simulink model "FSM"  (R2024b)
settings: Solver=VariableStepAuto  StartTime=0.0  StopTime=10.0  RelTol=1e-3
settings Model: Creator=leon-  LastModifiedBy=leon-

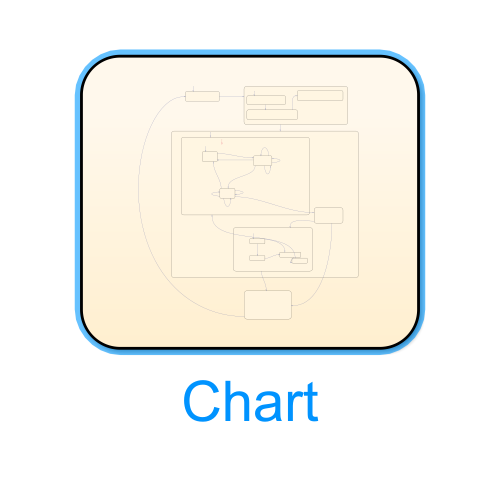
[thumbnail: Simulink's stored preview of the top-level diagram]
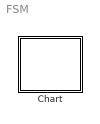
== system FSM ==
  Chart : Stateflow chart  TreatAsAtomicUnit=on

== stateflow chart FSM/Chart ==
  state Difficulty_Selection
    state Selected_Difficulty
      display_line1 = 'Selected Diff:';
      display_line2 = ['Level: ' num2str(difficulty_value)];
    state Inital_Difficulty
      display_line1 = "Difficuly";
      display_line2 = "Selection";
    state Change_Difficulty
      display_line1 = "Press Red: Change";
      display_line2 = "Press Blue: Start";
    (default) -> Inital_Difficulty : {timer = 0}
    Change_Difficulty -> Selected_Difficulty : [red_button]{changeLevel()}
    Inital_Difficulty -> Change_Difficulty : [timer > 3]
  state Idle
    display_line1="Reload and Press";
    display_line2="Button to Start";
  state In_Game
    state Human_Turn
      display_line1 = "Waiting for";
      display_line2 = "your Move";
      state Initial_IR
      state Triggered_IR
        triggered_IR = IR;
      state Wait_IR
      (default) -> Initial_IR
      Triggered_IR -> Triggered_IR [order 2] : [IR~=triggered_IR && ~timer_2]{timer_2 = 0}
      Initial_IR -> Triggered_IR : [IR]{timer_1 = 0}
      Triggered_IR -> Triggered_IR [order 4] : [IR~=triggered_IR && timer_2<0.01]
      Triggered_IR -> Initial_IR [order 1] : [IR~=triggered_IR] && timer_2=>0.01
      Wait_IR -> Initial_IR [order 3] : [IR~=triggered_IR] && timer_2=>0.01
      Triggered_IR -> Wait_IR [order 3] : [timer_1 > 0.02]{timer_1 = 0}
      Triggered_IR -> Triggered_IR [order 5] : [IR == triggered_IR]{~timer_2}
      Wait_IR -> Wait_IR [order 1] : [IR~=triggered_IR && ~timer_2]{timer_2 = 0}
      Wait_IR -> Wait_IR [order 4] : [IR == triggered_IR]{~timer_2}
      Wait_IR -> Wait_IR [order 2] : [IR~=triggered_IR && timer_2<0.01]
    state Game_Engine
      display_line1 = "Computing";
      display_line2 = "AI Move";
      updateBoard(human_col);
      AI_col = getBestMove();
    state AI_Turn
      display_line1 = "Machine executes";
      display_line2 = "Move";
      state Move_to_Mag
        motor_to_mag(AI_col)
      state Positioning
      state Initial_Move_to_Mag
        motor(dir = -1, speed = 10);
      state Move_to_AI_col
        motor_to_col(AI_col);
      (default) -> Positioning
      Move_to_AI_col -> Move_to_Mag : [complete]{~electromagnet}
      Positioning -> Move_to_AI_col [order 2] : [limit_switch1]{electromagnet}
      Positioning -> Initial_Move_to_Mag [order 1] : [~limit_switch1]
      Initial_Move_to_Mag -> Move_to_AI_col : [limit_switch1]{elecromagnet}
    (default) -> Human_Turn
    Wait_IR -> Game_Engine [order 5] : [timer_1 > 2]{human_col = triggered_IR}
    Move_to_Mag -> Human_Turn : [limit_switch1]
    Game_Engine -> AI_Turn [order 2] : [complete]
  state Game_Finish
    if (winner == "Draw") {
    display_line1 = "It's a Draw!";
    display_line2 = "";}
    else {
    display_line1 = "The winner is";
    display_line2 = winner;}
  (default) -> Idle
  Game_Finish -> Idle : [red_button || blue_button]
  Idle -> Difficulty_Selection : [red_button || blue_button]
  Difficulty_Selection -> In_Game : [blue_button]
  Game_Engine -> Game_Finish [order 1] : [is_winning_move(board, 2)]{winner = "You"}
  AI_Turn -> Game_Finish [order 1] : [is_winning_move(board, 1)]{winner = "Machine"}
  AI_Turn -> Game_Finish [order 2] : [is_draw(board)]{winner = "Draw"}
  data: IR parameter; timer local
